simulink model "W04_P1_pid_step"  (R2024b)
settings: Solver=ode4  StartTime=0.0  StopTime=10  FixedStep=0.001  RelTol=1e-3
values from neighbouring files (symbols this model uses):
  Kd = 400    [W04_heading_sign.m]    (also in W04_pole_place.m = G{i,3}; W04_setup.m = 0)
  Ki = fieldOr(fixed, 'Ki_u', evalin('base','Ki_u'))    [W04_pid_compare.m]    (also in W04_setup.m = 0)
  Kp = 800    [W04_heading_sign.m]    (also in W04_pid_compare.m = fieldOr(fixed, 'Kp_u', evalin('base','Kp_u')); W04_pole_place.m = G{i,2}; W04_setup.m = 10)
  Nf = 20    [W04_setup.m]
  plant_den = [1 2 2]    [W04_setup.m]
  plant_num = 1    [W04_setup.m]
libraries: slpidlib x1
settings Model: Creator=admin  LastModifiedBy=admin

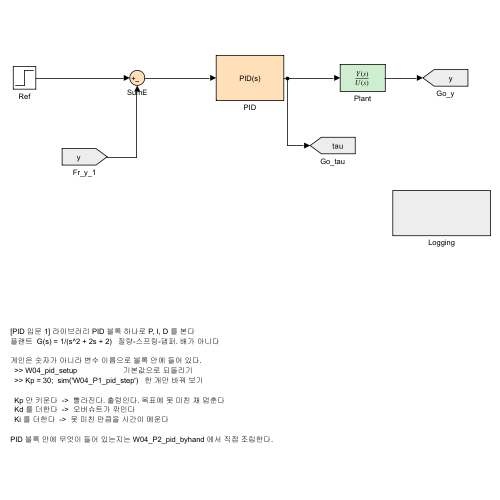
[thumbnail: Simulink's stored preview of the top-level diagram]
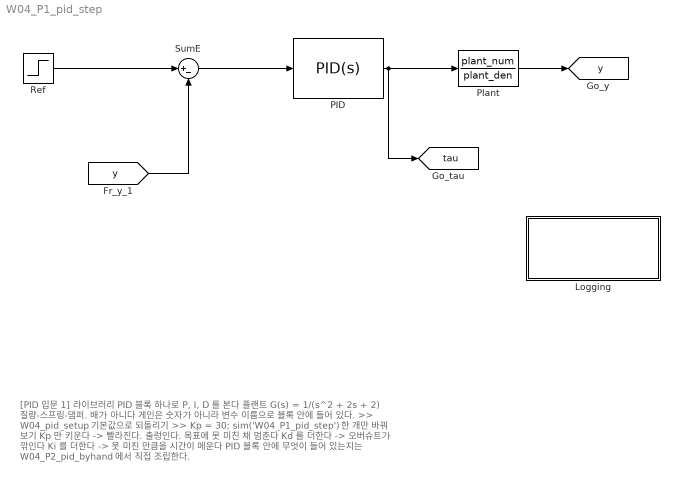
== system W04_P1_pid_step ==
  note: [PID 입문 1] 라이브러리 PID 블록 하나로 P, I, D 를 본다
      | 플랜트  G(s) = 1/(s^2 + 2s + 2)   질량-스프링-댐퍼. 배가 아니다
      |
      | 게인은 숫자가 아니라 변수 이름으로 블록 안에 들어 있다.
      |   >> W04_pid_setup                      기본값으로 되돌리기
      |   >> Kp = 30;  sim('W04_P1_pid_step')   한 개만 바꿔 보기
      |
      |   Kp 만 키운다  ->  빨라진다. 출렁인다. 목표에 못 미친 채 멈춘다
      |   Kd 를 더한다  ->  오버슈트가 깎인다
      |   Ki 를 더한다  ->  못 미친 만큼을 시간이 메운다
      |
      | PID 블록 안에 무엇이 들어 있는지는 W04_P2_pid_byhand 에서 직접 조립한다.
  Logging : Subsystem
  PID : slpidlib/PID Controller  Controller=PID  Form=Parallel  TimeDomain=Continuous-time  UseExternalTs=off  SampleTime=-1  IntegratorMethod=Forward Euler  FilterMethod=Forward Euler  ControllerParametersSource=internal  P=Kp  I=Ki  UseKiTs=off  D=Kd  UseExternalDerivativeSource=off  N=Nf  UseFilter=on  TunerSelectOption=Transfer Function Based (PID Tuner App)  InitialConditionSource=internal  InitialConditionForIntegrator=0  InitialConditionForFilter=0  DifferentiatorICPrevScaledInput=0  ExternalReset=none  TrackingMode=off  Kt=1  LimitOutput=off  SatLimitsSource=internal  UpperSaturationLimit=inf  LowerSaturationLimit=-inf  LinearizeAsGain=on  AntiWindupMode=none  Kb=1  LimitIntegrator=off  UpperIntegratorSaturationLimit=inf  LowerIntegratorSaturationLimit=-inf  POutMin=[]  POutMax=[]  IOutMin=[]  IOutMax=[]  DOutMin=[]  DOutMax=[]  NOutMin=[]  NOutMax=[]  SumOutMin=[]  SumOutMax=[]  SaturationOutMin=[]  SaturationOutMax=[]  PParamMin=[]  PParamMax=[]  IParamMin=[]  IParamMax=[]  DParamMin=[]  DParamMax=[]  NParamMin=[]  NParamMax=[]  KbParamMin=[]  KbParamMax=[]  KtParamMin=[]  KtParamMax=[]  KbOutMin=[]  KbOutMax=[]  KtOutMin=[]  KtOutMax=[]  IntegratorOutMin=[]  IntegratorOutMax=[]  FilterOutMin=[]  FilterOutMax=[]  SumI1OutMin=[]  SumI1OutMax=[]  SumI2OutMin=[]  SumI2OutMax=[]  SumI3OutMin=[]  SumI3OutMax=[]  SumI4OutMin=[]  SumI4OutMax=[]  SumDOutMin=[]  SumDOutMax=[]  DifferentiatorOutMin=[]  DifferentiatorOutMax=[]  FilterDiffOutCoefMin=[]  FilterDiffOutCoefMax=[]  ReciprocalOutMin=[]  ReciprocalOutMax=[]  SumDenOutMin=[]  SumDenOutMax=[]  SumNumOutMin=[]  SumNumOutMax=[]  DivideOutMin=[]  DivideOutMax=[]  UdiffTsProdOutMin=[]  UdiffTsProdOutMax=[]  NTsProdOutMin=[]  NTsProdOutMax=[]  UintegralTsProdOutMin=[]  UintegralTsProdOutMax=[]  UngainTsProdOutMin=[]  UngainTsProdOutMax=[]  ClampingZeroOutDataTypeStr=Inherit: Inherit via back propagation  ClampingZeroOutMin=[]  ClampingZeroOutMax=[]  FilterDenConstantOutDataTypeStr=Inherit: Inherit via back propagation  FilterDenConstantOutMin=[]  FilterDenConstantOutMax=[]  PCopyOutDataTypeStr=Inherit: Inherit via back propagation  PCopyOutMin=[]  PCopyOutMax=[]  NCopyOutDataTypeStr=Inherit: Inherit via back propagation  NCopyOutMin=[]  NCopyOutMax=[]  IntegratorContinuousStateAttributes=''  IntegratorStateMustResolveToSignalObject=off  IntegratorRTWStateStorageClass=Auto  FilterContinuousStateAttributes=''  FilterStateMustResolveToSignalObject=off  FilterRTWStateStorageClass=Auto  ParallelPVariant=InternalParameters  IdealPVariant=Disabled  IVariant=InternalParameters  DVariant=InternalParameters  IntegratorVariant=Continuous  SatVariant=Disabled  AWVariant=Passthrough  PCopyVariant=Disabled  TRVariant=Disabled  FdbkBlocksVariant=Forward  IdealPFdbkVariant=Disabled  SatFdbkVariant=Disabled  DerivativeFilterVariant=ContFilter  NVariant=InternalParameters  NCopyVariant=Disabled  FilterICVariant=InternalICsFilter  IntegratorICVariant=InternalICs  ExternalResetVariant=Disabled  TRSumVariant=Passthrough  SumFdbkVariant=Disabled  SumVariant=Sum_PID  TsampFilterVariant=InternalTs  TsampNgainVariant=Passthrough  TsampIntegralVariant=Disabled_SignalSpec  ExternalSaturationOutDataTypeStr=Inherit: Same as second input  DerivativeSourceVariant=ErrorSignal  PreIntVariant=InternalPreInt
  Plant : TransferFcn  Numerator=plant_num  Denominator=plant_den
  Ref : Step  SampleTime=0
  SumE : Sum  Inputs=|+-
  tag scope: tau=global, y=global
  wires:
  Ref/1 -> SumE/1
  SumE/1 -> PID/1
  PID/1 -> Plant/1, [tau]
  Plant/1 -> [y]
  [y] -> SumE/2

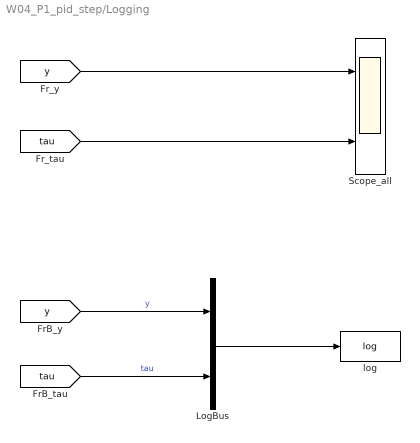
== system W04_P1_pid_step/Logging ==
  LogBus : BusCreator  Inputs=2
  Scope_all : Scope  NumInputPorts=2
  log : ToWorkspace  VariableName=log  SaveFormat=Timeseries  SampleTime=-1
  wires:
  [y] -> Scope_all/1
  [tau] -> Scope_all/2
  [y] -> LogBus/1  "y"
  [tau] -> LogBus/2  "tau"
  LogBus/1 -> log/1
